simulink model "State"  (R2019b)
settings: Solver=VariableStepAuto  StartTime=0.0  StopTime=10.0  RelTol=1e-3
settings Model: Creator=Lenovo  LastModifiedBy=Lenovo
settings OptimizationCC: DefaultParameterBehavior=Inlined

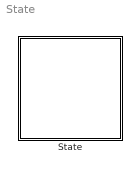
== system State ==
  State : Stateflow chart  BlockKeywords=__PRM__SERIALIZED__DATA__:Stateflow Chart,Stateflow Diagram  TreatAsAtomicUnit=on

== stateflow chart State/State ==
  state On
  state OFF
  state RESET
  (default) -> On
  RESET -> On
  OFF -> On [order 1]
  On -> OFF
  OFF -> RESET [order 2]
